simulink model "MIL_ASW"  (R2019b)
settings: Solver=FixedStepDiscrete  StartTime=0.0  StopTime=2  FixedStep=0.001  RelTol=1e-3  EnableMultiTasking=on
model workspace (MAT data in the model file):
  AccPedlCanVal = Simulink.Signal
  AccPedlCanVal.Description = 'the raw value of Engine Throttle from CAN, 0-255'
  AccPedlCanVal.DataType = 'uint8'
  AccPedlCanVal.Dimensions = -1
  AccPedlCanVal.DimensionsMode = 'auto'
  AccPedlCanVal.Complexity = 'auto'
  AccPedlCanVal.SampleTime = -1
  AccPedlCanVal.SamplingMode = 'auto'
  AccPedlVal = Simulink.Signal
  AccPedlVal.Description = 'the value of Engine Throttle percentage, 0-100'
  AccPedlVal.DataType = 'uint8'
  AccPedlVal.Dimensions = -1
  AccPedlVal.DimensionsMode = 'auto'
  AccPedlVal.Complexity = 'auto'
  AccPedlVal.SampleTime = -1
  AccPedlVal.SamplingMode = 'auto'
  BrkPedlCanVal = Simulink.Signal
  BrkPedlCanVal.Description = 'the raw value of Brake from CAN, 0-255'
  BrkPedlCanVal.DataType = 'uint8'
  BrkPedlCanVal.Dimensions = -1
  BrkPedlCanVal.DimensionsMode = 'auto'
  BrkPedlCanVal.Complexity = 'auto'
  BrkPedlCanVal.SampleTime = -1
  BrkPedlCanVal.SamplingMode = 'auto'
  BrkPedlVal = Simulink.Signal
  BrkPedlVal.Description = 'the value of Brake Pedal percentage, 0-100'
  BrkPedlVal.DataType = 'uint8'
  BrkPedlVal.Dimensions = -1
  BrkPedlVal.DimensionsMode = 'auto'
  BrkPedlVal.Complexity = 'auto'
  BrkPedlVal.SampleTime = -1
  BrkPedlVal.SamplingMode = 'auto'
  Cal1 = Simulink.Parameter
  Cal1.Value = 100
  Cal1.DataType = 'uint16'
  Cal1.Dimensions = [1 1]
  Cal10 = Simulink.Parameter
  Cal10.Value = 10
  Cal10.DataType = 'uint16'
  Cal10.Dimensions = [1 1]
  Cal11 = Simulink.Parameter
  Cal11.Value = 50
  Cal11.DataType = 'uint16'
  Cal11.Dimensions = [1 1]
  Cal12 = Simulink.Parameter
  Cal12.Value = 50
  Cal12.DataType = 'int16'
  Cal12.Dimensions = [1 1]
  Cal2 = Simulink.Parameter
  Cal2.Value = 10
  Cal2.DataType = 'uint16'
  Cal2.Dimensions = [1 1]
  Cal3 = Simulink.Parameter
  Cal3.Value = 200
  Cal3.DataType = 'uint16'
  Cal3.Dimensions = [1 1]
  Cal4 = Simulink.Parameter
  Cal4.Value = 50
  Cal4.DataType = 'int16'
  Cal4.Dimensions = [1 1]
  Cal5 = Simulink.Parameter
  Cal5.Value = 100
  Cal5.DataType = 'uint16'
  Cal5.Dimensions = [1 1]
  Cal6 = Simulink.Parameter
  Cal6.Value = 10
  Cal6.DataType = 'uint16'
  Cal6.Dimensions = [1 1]
  Cal7 = Simulink.Parameter
  Cal7.Value = 50
  Cal7.DataType = 'uint16'
  Cal7.Dimensions = [1 1]
  Cal8 = Simulink.Parameter
  Cal8.Value = 50
  Cal8.DataType = 'int16'
  Cal8.Dimensions = [1 1]
  Cal9 = Simulink.Parameter
  Cal9.Value = 100
  Cal9.DataType = 'uint16'
  Cal9.Dimensions = [1 1]
  Clu1Act = Simulink.Signal
  Clu1Act.DataType = 'uint8'
  Clu1Act.Dimensions = -1
  Clu1Act.DimensionsMode = 'auto'
  Clu1Act.Complexity = 'auto'
  Clu1Act.SampleTime = -1
  Clu1Act.SamplingMode = 'auto'
  Clu1PTar = Simulink.Signal
  Clu1PTar.DataType = 'uint16'
  Clu1PTar.Dimensions = -1
  Clu1PTar.DimensionsMode = 'auto'
  Clu1PTar.Complexity = 'auto'
  Clu1PTar.SampleTime = -1
  Clu1PTar.SamplingMode = 'auto'
  Clu1Req = Simulink.Signal
  Clu1Req.DataType = 'uint8'
  Clu1Req.Dimensions = -1
  Clu1Req.DimensionsMode = 'auto'
  Clu1Req.Complexity = 'auto'
  Clu1Req.SampleTime = -1
  Clu1Req.SamplingMode = 'auto'
  Clu1Req.InitialValue = '0'
  Clu1TqTar = Simulink.Signal
  Clu1TqTar.DataType = 'uint16'
  Clu1TqTar.Dimensions = -1
  Clu1TqTar.DimensionsMode = 'auto'
  Clu1TqTar.Complexity = 'auto'
  Clu1TqTar.SampleTime = -1
  Clu1TqTar.SamplingMode = 'auto'
  Clu2Act = Simulink.Signal
  Clu2Act.DataType = 'uint8'
  Clu2Act.Dimensions = -1
  Clu2Act.DimensionsMode = 'auto'
  Clu2Act.Complexity = 'auto'
  Clu2Act.SampleTime = -1
  Clu2Act.SamplingMode = 'auto'
  Clu2PTar = Simulink.Signal
  Clu2PTar.DataType = 'uint16'
  Clu2PTar.Dimensions = -1
  Clu2PTar.DimensionsMode = 'auto'
  Clu2PTar.Complexity = 'auto'
  Clu2PTar.SampleTime = -1
  Clu2PTar.SamplingMode = 'auto'
  Clu2Req = Simulink.Signal
  Clu2Req.DataType = 'uint8'
  Clu2Req.Dimensions = -1
  Clu2Req.DimensionsMode = 'auto'
  Clu2Req.Complexity = 'auto'
  Clu2Req.SampleTime = -1
  Clu2Req.SamplingMode = 'auto'
  Clu2Req.InitialValue = '0'
  Clu2TqTar = Simulink.Signal
  Clu2TqTar.DataType = 'uint16'
  Clu2TqTar.Dimensions = -1
  Clu2TqTar.DimensionsMode = 'auto'
  Clu2TqTar.Complexity = 'auto'
  Clu2TqTar.SampleTime = -1
  Clu2TqTar.SamplingMode = 'auto'
  CluKissPtPLnch = Simulink.Parameter
  CluKissPtPLnch.Value = 2200
  CluKissPtPLnch.DataType = 'uint16'
  CluKissPtPLnch.Dimensions = [1 1]
  CluOilTRawVal = Simulink.Signal
  CluOilTRawVal.Description = 'the raw value of Clutch oil temperature sensor, 0-255'
  CluOilTRawVal.DataType = 'uint16'
  CluOilTRawVal.Dimensions = -1
  CluOilTRawVal.DimensionsMode = 'auto'
  CluOilTRawVal.Complexity = 'auto'
  CluOilTRawVal.SampleTime = -1
  CluOilTRawVal.SamplingMode = 'auto'
  CluOilTVal = Simulink.Signal
  CluOilTVal.Description = 'the value of Clutch oil temperature'
  CluOilTVal.DataType = 'uint16'
  CluOilTVal.Dimensions = -1
  CluOilTVal.DimensionsMode = 'auto'
  CluOilTVal.Complexity = 'auto'
  CluOilTVal.SampleTime = -1
  CluOilTVal.SamplingMode = 'auto'
  CluOpenTqRatMax = Simulink.Parameter
  CluOpenTqRatMax.Value = 100
  CluOpenTqRatMax.DataType = 'uint16'
  CluOpenTqRatMax.Dimensions = [1 1]
  CluPMap = Simulink.Parameter
  CluPMap.Value = [0 1300 9000]
  CluPMap.DataType = 'uint16'
  CluPMap.Dimensions = [1 3]
  CluPMax = Simulink.Parameter
  CluPMax.Value = 600
  CluPMax.DataType = 'uint16'
  CluPMax.Dimensions = [1 1]
  CluPMaxGear1 = Simulink.Parameter
  CluPMaxGear1.Value = 4000
  CluPMaxGear1.DataType = 'uint16'
  CluPMaxGear1.Dimensions = [1 1]
  CluPMaxGear2 = Simulink.Parameter
  CluPMaxGear2.Value = 4500
  CluPMaxGear2.DataType = 'uint16'
  CluPMaxGear2.Dimensions = [1 1]
  CluPMaxGear3 = Simulink.Parameter
  CluPMaxGear3.Value = 5000
  CluPMaxGear3.DataType = 'uint16'
  CluPMaxGear3.Dimensions = [1 1]
  CluPMaxGear4 = Simulink.Parameter
  CluPMaxGear4.Value = 5500
  CluPMaxGear4.DataType = 'uint16'
  CluPMaxGear4.Dimensions = [1 1]
  CluPMaxGear5 = Simulink.Parameter
  CluPMaxGear5.Value = 6000
  CluPMaxGear5.DataType = 'uint16'
  CluPMaxGear5.Dimensions = [1 1]
  CluPMaxGear6 = Simulink.Parameter
  CluPMaxGear6.Value = 6000
  CluPMaxGear6.DataType = 'uint16'
  CluPMaxGear6.Dimensions = [1 1]
  CluPMaxGearR = Simulink.Parameter
  CluPMaxGearR.Value = 3500
  CluPMaxGearR.DataType = 'uint16'
  CluPMaxGearR.Dimensions = [1 1]
  CluPMin = Simulink.Parameter
  CluPMin.Value = 1300
  CluPMin.DataType = 'uint16'
  CluPMin.Dimensions = [1 1]
  CluPosnMax = Simulink.Parameter
  CluPosnMax.Value = 4550
  CluPosnMax.DataType = 'uint16'
  CluPosnMax.Dimensions = [1 1]
  CluSoln1IRawVal = Simulink.Signal
  CluSoln1IRawVal.DataType = 'uint16'
  CluSoln1IRawVal.Dimensions = -1
  CluSoln1IRawVal.DimensionsMode = 'auto'
  CluSoln1IRawVal.Complexity = 'auto'
  CluSoln1IRawVal.SampleTime = -1
  CluSoln1IRawVal.SamplingMode = 'auto'
  CluSoln1IReq = Simulink.Signal
  CluSoln1IReq.DataType = 'uint16'
  CluSoln1IReq.Dimensions = -1
  CluSoln1IReq.DimensionsMode = 'auto'
  CluSoln1IReq.Complexity = 'auto'
  CluSoln1IReq.SampleTime = -1
  CluSoln1IReq.SamplingMode = 'auto'
  CluSoln1IReqFlg = Simulink.Signal
  CluSoln1IReqFlg.DataType = 'uint8'
  CluSoln1IReqFlg.Dimensions = -1
  CluSoln1IReqFlg.DimensionsMode = 'auto'
  CluSoln1IReqFlg.Complexity = 'auto'
  CluSoln1IReqFlg.SampleTime = -1
  CluSoln1IReqFlg.SamplingMode = 'auto'
  CluSoln1IVal = Simulink.Signal
  CluSoln1IVal.DataType = 'uint16'
  CluSoln1IVal.Dimensions = -1
  CluSoln1IVal.DimensionsMode = 'auto'
  CluSoln1IVal.Complexity = 'auto'
  CluSoln1IVal.SampleTime = -1
  CluSoln1IVal.SamplingMode = 'auto'
  CluSoln1LineI = Simulink.Parameter
  CluSoln1LineI.Value = [0 200 400 600 800 950]
  CluSoln1LineI.DataType = 'uint16'
  CluSoln1LineI.Dimensions = [1 6]
  CluSoln1LineP = Simulink.Parameter
  CluSoln1LineP.Value = [0 1 2500 8850 15770 20000]
  CluSoln1LineP.DataType = 'uint16'
  CluSoln1LineP.Dimensions = [1 6]
  CluSoln1Pwm = Simulink.Signal
  CluSoln1Pwm.DataType = 'uint16'
  CluSoln1Pwm.Dimensions = -1
  CluSoln1Pwm.DimensionsMode = 'auto'
  CluSoln1Pwm.Complexity = 'auto'
  CluSoln1Pwm.SampleTime = -1
  CluSoln1Pwm.SamplingMode = 'auto'
  CluSoln2IRawVal = Simulink.Signal
  CluSoln2IRawVal.DataType = 'uint16'
  CluSoln2IRawVal.Dimensions = -1
  CluSoln2IRawVal.DimensionsMode = 'auto'
  CluSoln2IRawVal.Complexity = 'auto'
  CluSoln2IRawVal.SampleTime = -1
  CluSoln2IRawVal.SamplingMode = 'auto'
  CluSoln2IReq = Simulink.Signal
  CluSoln2IReq.DataType = 'uint16'
  CluSoln2IReq.Dimensions = -1
  CluSoln2IReq.DimensionsMode = 'auto'
  CluSoln2IReq.Complexity = 'auto'
  CluSoln2IReq.SampleTime = -1
  CluSoln2IReq.SamplingMode = 'auto'
  CluSoln2IReqFlg = Simulink.Signal
  CluSoln2IReqFlg.DataType = 'uint8'
  CluSoln2IReqFlg.Dimensions = -1
  CluSoln2IReqFlg.DimensionsMode = 'auto'
  CluSoln2IReqFlg.Complexity = 'auto'
  CluSoln2IReqFlg.SampleTime = -1
  CluSoln2IReqFlg.SamplingMode = 'auto'
  CluSoln2IVal = Simulink.Signal
  CluSoln2IVal.DataType = 'uint16'
  CluSoln2IVal.Dimensions = -1
  CluSoln2IVal.DimensionsMode = 'auto'
  CluSoln2IVal.Complexity = 'auto'
  CluSoln2IVal.SampleTime = -1
  CluSoln2IVal.SamplingMode = 'auto'
  CluSoln2LineI = Simulink.Parameter
  CluSoln2LineI.Value = [0 200 400 600 800 950]
  CluSoln2LineI.DataType = 'uint16'
  CluSoln2LineI.Dimensions = [1 6]
  CluSoln2LineP = Simulink.Parameter
  CluSoln2LineP.Value = [0 1 2500 8850 15770 20000]
  CluSoln2LineP.DataType = 'uint16'
  CluSoln2LineP.Dimensions = [1 6]
  CluSoln2Pwm = Simulink.Signal
  CluSoln2Pwm.DataType = 'uint16'
  CluSoln2Pwm.Dimensions = -1
  CluSoln2Pwm.DimensionsMode = 'auto'
  CluSoln2Pwm.Complexity = 'auto'
  CluSoln2Pwm.SampleTime = -1
  CluSoln2Pwm.SamplingMode = 'auto'
  CluTqMap = Simulink.Parameter
  CluTqMap.Value = [0 1 35000]
  CluTqMap.DataType = 'uint16'
  CluTqMap.Dimensions = [1 3]
  CrnkSpdRawVal = Simulink.Signal
  CrnkSpdRawVal.Description = 'the raw value of the frequency of crank shaft signal, Hz'
  CrnkSpdRawVal.DataType = 'uint16'
  CrnkSpdRawVal.Dimensions = -1
  CrnkSpdRawVal.DimensionsMode = 'auto'
  CrnkSpdRawVal.Complexity = 'auto'
  CrnkSpdRawVal.SampleTime = -1
  CrnkSpdRawVal.SamplingMode = 'auto'
  CrnkSpdVal = Simulink.Signal
  CrnkSpdVal.Description = 'the value of enigne crank shaft speed, rpm'
  CrnkSpdVal.DataType = 'uint16'
  CrnkSpdVal.Dimensions = -1
  CrnkSpdVal.DimensionsMode = 'auto'
  CrnkSpdVal.Complexity = 'auto'
  CrnkSpdVal.SampleTime = -1
  CrnkSpdVal.SamplingMode = 'auto'
  Drive_Intensity_Fuzzy.name = 'Launch_Intensity_Fuzzy'
  Drive_Intensity_Fuzzy.type = 'mamdani'
  Drive_Intensity_Fuzzy.andMethod = 'min'
  Drive_Intensity_Fuzzy.orMethod = 'max'
  Drive_Intensity_Fuzzy.defuzzMethod = 'centroid'
  Drive_Intensity_Fuzzy.impMethod = 'min'
  Drive_Intensity_Fuzzy.aggMethod = 'max'
  Drive_Intensity_Fuzzy.input(1).name = 'Pedl'
  Drive_Intensity_Fuzzy.input(1).range = [0 100]
  Drive_Intensity_Fuzzy.input(1).mf(1).name = 'VS'
  Drive_Intensity_Fuzzy.input(1).mf(1).type = 'trimf'
  Drive_Intensity_Fuzzy.input(1).mf(1).params = [0 0 25]
  Drive_Intensity_Fuzzy.input(1).mf(2).name = 'S'
  Drive_Intensity_Fuzzy.input(1).mf(2).type = 'trimf'
  Drive_Intensity_Fuzzy.input(1).mf(2).params = [0 25 50]
  Drive_Intensity_Fuzzy.input(1).mf(3).name = 'M'
  Drive_Intensity_Fuzzy.input(1).mf(3).type = 'trimf'
  Drive_Intensity_Fuzzy.input(1).mf(3).params = [25 50 75]
  Drive_Intensity_Fuzzy.input(1).mf(4).name = 'B'
  Drive_Intensity_Fuzzy.input(1).mf(4).type = 'trimf'
  Drive_Intensity_Fuzzy.input(1).mf(4).params = [50 75 100]
  Drive_Intensity_Fuzzy.input(1).mf(5).name = 'VB'
  Drive_Intensity_Fuzzy.input(1).mf(5).type = 'trimf'
  Drive_Intensity_Fuzzy.input(1).mf(5).params = [75 100 110]
  Drive_Intensity_Fuzzy.input(2).name = 'dPedl'
  Drive_Intensity_Fuzzy.input(2).range = [-300 300]
  Drive_Intensity_Fuzzy.input(2).mf(1).name = 'NB'
  Drive_Intensity_Fuzzy.input(2).mf(1).type = 'trimf'
  Drive_Intensity_Fuzzy.input(2).mf(1).params = [-300 -300 -100]
  Drive_Intensity_Fuzzy.input(2).mf(2).name = 'NS'
  Drive_Intensity_Fuzzy.input(2).mf(2).type = 'trimf'
  Drive_Intensity_Fuzzy.input(2).mf(2).params = [-300 -100 0]
  Drive_Intensity_Fuzzy.input(2).mf(3).name = 'Z'
  Drive_Intensity_Fuzzy.input(2).mf(3).type = 'trimf'
  Drive_Intensity_Fuzzy.input(2).mf(3).params = [-100 0 100]
  Drive_Intensity_Fuzzy.input(2).mf(4).name = 'PS'
  Drive_Intensity_Fuzzy.input(2).mf(4).type = 'trimf'
  Drive_Intensity_Fuzzy.input(2).mf(4).params = [0 100 200]
  Drive_Intensity_Fuzzy.input(2).mf(5).name = 'PM'
  Drive_Intensity_Fuzzy.input(2).mf(5).type = 'trimf'
  Drive_Intensity_Fuzzy.input(2).mf(5).params = [100 200 300]
  Drive_Intensity_Fuzzy.input(2).mf(6).name = 'PB'
  Drive_Intensity_Fuzzy.input(2).mf(6).type = 'trimf'
  Drive_Intensity_Fuzzy.input(2).mf(6).params = [200 300 350]
  Drive_Intensity_Fuzzy.output.name = 'Inten'
  Drive_Intensity_Fuzzy.output.range = [0 100]
  Drive_Intensity_Fuzzy.output.mf(1).name = 'VS'
  Drive_Intensity_Fuzzy.output.mf(1).type = 'trimf'
  Drive_Intensity_Fuzzy.output.mf(1).params = [0 0 25]
  Drive_Intensity_Fuzzy.output.mf(2).name = 'S'
  Drive_Intensity_Fuzzy.output.mf(2).type = 'trimf'
  Drive_Intensity_Fuzzy.output.mf(2).params = [0 25 50]
  Drive_Intensity_Fuzzy.output.mf(3).name = 'M'
  Drive_Intensity_Fuzzy.output.mf(3).type = 'trimf'
  Drive_Intensity_Fuzzy.output.mf(3).params = [25 50 75]
  Drive_Intensity_Fuzzy.output.mf(4).name = 'F'
  Drive_Intensity_Fuzzy.output.mf(4).type = 'trimf'
  Drive_Intensity_Fuzzy.output.mf(4).params = [50 75 100]
  Drive_Intensity_Fuzzy.output.mf(5).name = 'VF'
  Drive_Intensity_Fuzzy.output.mf(5).type = 'trimf'
  Drive_Intensity_Fuzzy.output.mf(5).params = [75 100 110]
  Drive_Intensity_Fuzzy.rule(1).antecedent = [1 1]
  Drive_Intensity_Fuzzy.rule(1).consequent = 1
  Drive_Intensity_Fuzzy.rule(1).weight = 1
  Drive_Intensity_Fuzzy.rule(1).connection = 1
  Drive_Intensity_Fuzzy.rule(2).antecedent = [1 2]
  Drive_Intensity_Fuzzy.rule(2).consequent = 1
  Drive_Intensity_Fuzzy.rule(2).weight = 1
  Drive_Intensity_Fuzzy.rule(2).connection = 1
  Drive_Intensity_Fuzzy.rule(3).antecedent = [1 3]
  Drive_Intensity_Fuzzy.rule(3).consequent = 1
  Drive_Intensity_Fuzzy.rule(3).weight = 1
  Drive_Intensity_Fuzzy.rule(3).connection = 1
  Drive_Intensity_Fuzzy.rule(4).antecedent = [1 4]
  Drive_Intensity_Fuzzy.rule(4).consequent = 2
  Drive_Intensity_Fuzzy.rule(4).weight = 1
  Drive_Intensity_Fuzzy.rule(4).connection = 1
  Drive_Intensity_Fuzzy.rule(5).antecedent = [1 5]
  Drive_Intensity_Fuzzy.rule(5).consequent = 3
  Drive_Intensity_Fuzzy.rule(5).weight = 1
  Drive_Intensity_Fuzzy.rule(5).connection = 1
  Drive_Intensity_Fuzzy.rule(6).antecedent = [1 6]
  Drive_Intensity_Fuzzy.rule(6).consequent = 4
  Drive_Intensity_Fuzzy.rule(6).weight = 1
  Drive_Intensity_Fuzzy.rule(6).connection = 1
  Drive_Intensity_Fuzzy.rule(7).antecedent = [2 1]
  Drive_Intensity_Fuzzy.rule(7).consequent = 1
  Drive_Intensity_Fuzzy.rule(7).weight = 1
  Drive_Intensity_Fuzzy.rule(7).connection = 1
  Drive_Intensity_Fuzzy.rule(8).antecedent = [2 2]
  Drive_Intensity_Fuzzy.rule(8).consequent = 2
  Drive_Intensity_Fuzzy.rule(8).weight = 1
  Drive_Intensity_Fuzzy.rule(8).connection = 1
  Drive_Intensity_Fuzzy.rule(9).antecedent = [2 3]
  Drive_Intensity_Fuzzy.rule(9).consequent = 2
  Drive_Intensity_Fuzzy.rule(9).weight = 1
  Drive_Intensity_Fuzzy.rule(9).connection = 1
  Drive_Intensity_Fuzzy.rule(10).antecedent = [2 4]
  Drive_Intensity_Fuzzy.rule(10).consequent = 3
  Drive_Intensity_Fuzzy.rule(10).weight = 1
  Drive_Intensity_Fuzzy.rule(10).connection = 1
  Drive_Intensity_Fuzzy.rule(11).antecedent = [2 5]
  Drive_Intensity_Fuzzy.rule(11).consequent = 4
  Drive_Intensity_Fuzzy.rule(11).weight = 1
  Drive_Intensity_Fuzzy.rule(11).connection = 1
  Drive_Intensity_Fuzzy.rule(12).antecedent = [2 6]
  Drive_Intensity_Fuzzy.rule(12).consequent = 4
  Drive_Intensity_Fuzzy.rule(12).weight = 1
  Drive_Intensity_Fuzzy.rule(12).connection = 1
  Drive_Intensity_Fuzzy.rule(13).antecedent = [3 1]
  Drive_Intensity_Fuzzy.rule(13).consequent = 1
  Drive_Intensity_Fuzzy.rule(13).weight = 1
  Drive_Intensity_Fuzzy.rule(13).connection = 1
  Drive_Intensity_Fuzzy.rule(14).antecedent = [3 2]
  Drive_Intensity_Fuzzy.rule(14).consequent = 2
  Drive_Intensity_Fuzzy.rule(14).weight = 1
  Drive_Intensity_Fuzzy.rule(14).connection = 1
  Drive_Intensity_Fuzzy.rule(15).antecedent = [3 3]
  Drive_Intensity_Fuzzy.rule(15).consequent = 3
  Drive_Intensity_Fuzzy.rule(15).weight = 1
  Drive_Intensity_Fuzzy.rule(15).connection = 1
  Drive_Intensity_Fuzzy.rule(16).antecedent = [3 4]
  Drive_Intensity_Fuzzy.rule(16).consequent = 4
  Drive_Intensity_Fuzzy.rule(16).weight = 1
  Drive_Intensity_Fuzzy.rule(16).connection = 1
  Drive_Intensity_Fuzzy.rule(17).antecedent = [3 5]
  Drive_Intensity_Fuzzy.rule(17).consequent = 5
  Drive_Intensity_Fuzzy.rule(17).weight = 1
  Drive_Intensity_Fuzzy.rule(17).connection = 1
  Drive_Intensity_Fuzzy.rule(18).antecedent = [3 6]
  Drive_Intensity_Fuzzy.rule(18).consequent = 5
  Drive_Intensity_Fuzzy.rule(18).weight = 1
  Drive_Intensity_Fuzzy.rule(18).connection = 1
  Drive_Intensity_Fuzzy.rule(19).antecedent = [4 1]
  Drive_Intensity_Fuzzy.rule(19).consequent = 1
  Drive_Intensity_Fuzzy.rule(19).weight = 1
  Drive_Intensity_Fuzzy.rule(19).connection = 1
  Drive_Intensity_Fuzzy.rule(20).antecedent = [4 2]
  Drive_Intensity_Fuzzy.rule(20).consequent = 2
  Drive_Intensity_Fuzzy.rule(20).weight = 1
  Drive_Intensity_Fuzzy.rule(20).connection = 1
  Drive_Intensity_Fuzzy.rule(21).antecedent = [4 3]
  Drive_Intensity_Fuzzy.rule(21).consequent = 4
  Drive_Intensity_Fuzzy.rule(21).weight = 1
  Drive_Intensity_Fuzzy.rule(21).connection = 1
  Drive_Intensity_Fuzzy.rule(22).antecedent = [4 4]
  Drive_Intensity_Fuzzy.rule(22).consequent = 4
  Drive_Intensity_Fuzzy.rule(22).weight = 1
  Drive_Intensity_Fuzzy.rule(22).connection = 1
  Drive_Intensity_Fuzzy.rule(23).antecedent = [4 5]
  Drive_Intensity_Fuzzy.rule(23).consequent = 5
  Drive_Intensity_Fuzzy.rule(23).weight = 1
  Drive_Intensity_Fuzzy.rule(23).connection = 1
  Drive_Intensity_Fuzzy.rule(24).antecedent = [4 6]
  Drive_Intensity_Fuzzy.rule(24).consequent = 5
  Drive_Intensity_Fuzzy.rule(24).weight = 1
  Drive_Intensity_Fuzzy.rule(24).connection = 1
  Drive_Intensity_Fuzzy.rule(25).antecedent = [5 1]
  Drive_Intensity_Fuzzy.rule(25).consequent = 1
  Drive_Intensity_Fuzzy.rule(25).weight = 1
  Drive_Intensity_Fuzzy.rule(25).connection = 1
  Drive_Intensity_Fuzzy.rule(26).antecedent = [5 2]
  Drive_Intensity_Fuzzy.rule(26).consequent = 2
  Drive_Intensity_Fuzzy.rule(26).weight = 1
  Drive_Intensity_Fuzzy.rule(26).connection = 1
  Drive_Intensity_Fuzzy.rule(27).antecedent = [5 3]
  Drive_Intensity_Fuzzy.rule(27).consequent = 5
  Drive_Intensity_Fuzzy.rule(27).weight = 1
  Drive_Intensity_Fuzzy.rule(27).connection = 1
  Drive_Intensity_Fuzzy.rule(28).antecedent = [5 4]
  Drive_Intensity_Fuzzy.rule(28).consequent = 5
  Drive_Intensity_Fuzzy.rule(28).weight = 1
  Drive_Intensity_Fuzzy.rule(28).connection = 1
  Drive_Intensity_Fuzzy.rule(29).antecedent = [5 5]
  Drive_Intensity_Fuzzy.rule(29).consequent = 5
  Drive_Intensity_Fuzzy.rule(29).weight = 1
  Drive_Intensity_Fuzzy.rule(29).connection = 1
  Drive_Intensity_Fuzzy.rule(30).antecedent = [5 6]
  Drive_Intensity_Fuzzy.rule(30).consequent = 5
  Drive_Intensity_Fuzzy.rule(30).weight = 1
  Drive_Intensity_Fuzzy.rule(30).connection = 1
  DrvIntenFzzy = Simulink.LookupTable
  DrvIntenFzzy.Table = Simulink.lookuptable.Table
  DrvIntenFzzy.Table.Value = [8  9  9  8  9  19  25  41  59  75; 9  20  21  21  21  31  36  52  61  75; 8  19  24  25  25  34  46  62  71  75; 9  19  24  25  34  45  59  67  76  76; 8  19  24  25  41  52  68  72  83  83; 8  19  24  25  48  59  75  81  91  92; 9  19  24  25  55  66  75  81  91  91; 8  19  24  25  56  75  75  81  91  92; 9  20  23  25  58  79  79  80  91  91; 8  19  24  25  55  91  92  91  91  92]
  DrvIntenFzzy.Table.Dimensions = [10 10]
  DrvIntenFzzy.Table.DataType = 'int16'
  DrvIntenFzzy.Table.FieldName = 'Table'
  DrvIntenFzzy.Breakpoints(1) = Simulink.lookuptable.Breakpoint
  DrvIntenFzzy.Breakpoints(1).Value = [0 11 22 33 44 56 67 78 89 100]
  DrvIntenFzzy.Breakpoints(1).TunableSizeName = 'N1'
  DrvIntenFzzy.Breakpoints(1).Dimensions = [1 10]
  DrvIntenFzzy.Breakpoints(1).DataType = 'int16'
  DrvIntenFzzy.Breakpoints(1).FieldName = 'BP1'
  DrvIntenFzzy.Breakpoints(2) = Simulink.lookuptable.Breakpoint
  DrvIntenFzzy.Breakpoints(2).Value = [-300 -233 -167 -100 -33 33 100 167 233 300]
  DrvIntenFzzy.Breakpoints(2).TunableSizeName = 'N2'
  DrvIntenFzzy.Breakpoints(2).Dimensions = [1 10]
  DrvIntenFzzy.Breakpoints(2).DataType = 'int16'
  DrvIntenFzzy.Breakpoints(2).FieldName = 'BP2'
  DrvIntenFzzy.SupportTunableSize = 0
  DrvIntenFzzy.StructTypeInfo = Simulink.lookuptable.StructTypeInfo
  DrvIntenFzzy.StructTypeInfo.Name = 'DrvIntenFzzyStruct'
  DrvIntenFzzy.StructTypeInfo.DataScope = 'Auto'
  EngNIdle = Simulink.Parameter
  EngNIdle.Value = 750
  EngNIdle.DataType = 'uint16'
  EngNIdle.Dimensions = [1 1]
  EngNIdleMin = Simulink.Parameter
  EngNIdleMin.Value = 400
  EngNIdleMin.DataType = 'uint16'
  EngNIdleMin.Dimensions = [1 1]
  EngSpdCanVal = Simulink.Signal
  EngSpdCanVal.Description = 'engine speed information from CAN bus'
  EngSpdCanVal.DataType = 'uint16'
  EngSpdCanVal.Dimensions = -1
  EngSpdCanVal.DimensionsMode = 'auto'
  EngSpdCanVal.Complexity = 'auto'
  EngSpdCanVal.SampleTime = -1
  EngSpdCanVal.SamplingMode = 'auto'
  EngThrCanVal = Simulink.Signal
  EngThrCanVal.Description = 'engine throttle opening information from CAN bus'
  EngThrCanVal.DataType = 'uint8'
  EngThrCanVal.Dimensions = -1
  EngThrCanVal.DimensionsMode = 'auto'
  EngThrCanVal.Complexity = 'auto'
  EngThrCanVal.SampleTime = -1
  EngThrCanVal.SamplingMode = 'auto'
  EngTqAdd = Simulink.Parameter
  EngTqAdd.Value = 2500
  EngTqAdd.DataType = 'uint16'
  EngTqAdd.Dimensions = [1 1]
  EngTqCanVal = Simulink.Signal
  EngTqCanVal.Description = 'engine torque information from CAN bus'
  EngTqCanVal.DataType = 'uint16'
  EngTqCanVal.Dimensions = -1
  EngTqCanVal.DimensionsMode = 'auto'
  EngTqCanVal.Complexity = 'auto'
  EngTqCanVal.SampleTime = -1
  EngTqCanVal.SamplingMode = 'auto'
  EngTqIntvFlg = Simulink.Signal
  EngTqIntvFlg.DataType = 'uint8'
  EngTqIntvFlg.Dimensions = -1
  EngTqIntvFlg.DimensionsMode = 'auto'
  EngTqIntvFlg.Complexity = 'auto'
  EngTqIntvFlg.SampleTime = -1
  EngTqIntvFlg.SamplingMode = 'auto'
  EngTqIntvRat = Simulink.Signal
  EngTqIntvRat.DataType = 'uint8'
  EngTqIntvRat.Dimensions = -1
  EngTqIntvRat.DimensionsMode = 'auto'
  EngTqIntvRat.Complexity = 'auto'
  EngTqIntvRat.SampleTime = -1
  EngTqIntvRat.SamplingMode = 'auto'
  EngTqMapExtChartc = Simulink.Parameter
  EngTqMapExtChartc.Value = [0 0 11817 21322 25300 28928 30352 32100 33708 35000 35000 35000 35000 35000 33732 32308 30670 26743 22827 14400 0]
  EngTqMapExtChartc.DataType = 'uint16'
  EngTqMapExtChartc.Dimensions = [1 21]
  EngTqMapSpdIndx = Simulink.Parameter
  EngTqMapSpdIndx.Value = [0 400 517 633 750 1107 1463 1820 2177 2533 2890 3247 3603 3960 4317 4673 5030 5387 5743 6100 6500]
  EngTqMapSpdIndx.DataType = 'uint16'
  EngTqMapSpdIndx.Dimensions = [1 21]
  EngTqMapThrtIndx = Simulink.Parameter
  EngTqMapThrtIndx.Value = [0 10 20 30 40 50 60 70 80 90 100]
  EngTqMapThrtIndx.DataType = 'uint8'
  EngTqMapThrtIndx.Dimensions = [1 11]
  EngTqMapTqMax = Simulink.Parameter
  EngTqMapTqMax.Value = [4179 4179 13259 23544 26944 29368 32550 33431 34042 34548 35000]
  EngTqMapTqMax.DataType = 'uint16'
  EngTqMapTqMax.Dimensions = [1 11]
  EngTqMaxNorm = Simulink.Parameter
  EngTqMaxNorm.Value = 35000
  EngTqMaxNorm.DataType = 'uint16'
  EngTqMaxNorm.Dimensions = [1 1]
  EngTqRef = Simulink.Parameter
  EngTqRef.Value = 250
  EngTqRef.DataType = 'uint16'
  EngTqRef.Dimensions = [1 1]
  EvenCluPRawVal = Simulink.Signal
  EvenCluPRawVal.Description = ' the raw value of Even Gear Clutch Pressure sensor, 0-255'
  EvenCluPRawVal.DataType = 'uint16'
  EvenCluPRawVal.Dimensions = -1
  EvenCluPRawVal.DimensionsMode = 'auto'
  EvenCluPRawVal.Complexity = 'auto'
  EvenCluPRawVal.SampleTime = -1
  EvenCluPRawVal.SamplingMode = 'auto'
  EvenCluPVal = Simulink.Signal
  EvenCluPVal.Description = 'the value of Even Gear Clutch Pressure sensor *10, Bar'
  EvenCluPVal.DataType = 'uint16'
  EvenCluPVal.Dimensions = -1
  EvenCluPVal.DimensionsMode = 'auto'
  EvenCluPVal.Complexity = 'auto'
  EvenCluPVal.SampleTime = -1
  EvenCluPVal.SamplingMode = 'auto'
  EvenInpSpdRawVal = Simulink.Signal
  EvenInpSpdRawVal.Description = 'the raw value of the frequency of even input shaft signal, Hz'
  EvenInpSpdRawVal.DataType = 'uint16'
  EvenInpSpdRawVal.Dimensions = -1
  EvenInpSpdRawVal.DimensionsMode = 'auto'
  EvenInpSpdRawVal.Complexity = 'auto'
  EvenInpSpdRawVal.SampleTime = -1
  EvenInpSpdRawVal.SamplingMode = 'auto'
  EvenInpSpdVal = Simulink.Signal
  EvenInpSpdVal.Description = 'the value of even input shaft speed, rpm'
  EvenInpSpdVal.DataType = 'uint16'
  EvenInpSpdVal.Dimensions = -1
  EvenInpSpdVal.DimensionsMode = 'auto'
  EvenInpSpdVal.Complexity = 'auto'
  EvenInpSpdVal.SampleTime = -1
  EvenInpSpdVal.SamplingMode = 'auto'
  FcnCallTime = Simulink.Parameter
  FcnCallTime.Value = 10
  FcnCallTime.DataType = 'uint8'
  FcnCallTime.Dimensions = [1 1]
  FinalRat = Simulink.Parameter
  FinalRat.Value = [428 285]
  FinalRat.DataType = 'uint16'
  FinalRat.Dimensions = [1 2]
  Fork1A = Simulink.Parameter
  Fork1A.Value = 1
  Fork1A.DataType = 'uint8'
  Fork1A.Dimensions = [1 1]
  Fork1Act = Simulink.Signal
  Fork1Act.DataType = 'uint8'
  Fork1Act.Dimensions = -1
  Fork1Act.DimensionsMode = 'auto'
  Fork1Act.Complexity = 'auto'
  Fork1Act.SampleTime = -1
  Fork1Act.SamplingMode = 'auto'
  Fork1B = Simulink.Parameter
  Fork1B.Value = 3
  Fork1B.DataType = 'uint8'
  Fork1B.Dimensions = [1 1]
  Fork1DeltaSpdTar = Simulink.Parameter
  Fork1DeltaSpdTar.Value = 20
  Fork1DeltaSpdTar.DataType = 'uint16'
  Fork1DeltaSpdTar.Dimensions = [1 1]
  Fork1MaxSpd1A = Simulink.Parameter
  Fork1MaxSpd1A.Value = 4400
  Fork1MaxSpd1A.DataType = 'uint16'
  Fork1MaxSpd1A.Dimensions = [1 1]
  Fork1MaxSpd1B = Simulink.Parameter
  Fork1MaxSpd1B.Value = 4400
  Fork1MaxSpd1B.DataType = 'uint16'
  Fork1MaxSpd1B.Dimensions = [1 1]
  Fork1MaxSpd2A = Simulink.Parameter
  Fork1MaxSpd2A.Value = 3400
  Fork1MaxSpd2A.DataType = 'uint16'
  Fork1MaxSpd2A.Dimensions = [1 1]
  Fork1MaxSpd2B = Simulink.Parameter
  Fork1MaxSpd2B.Value = 3400
  Fork1MaxSpd2B.DataType = 'uint16'
  Fork1MaxSpd2B.Dimensions = [1 1]
  Fork1PosnA = Simulink.Parameter
  Fork1PosnA.Value = 795
  Fork1PosnA.DataType = 'uint16'
  Fork1PosnA.Dimensions = [1 1]
  Fork1PosnB = Simulink.Parameter
  Fork1PosnB.Value = 249
  Fork1PosnB.DataType = 'uint16'
  Fork1PosnB.Dimensions = [1 1]
  Fork1PosnMaxSpd1A = Simulink.Parameter
  Fork1PosnMaxSpd1A.Value = 560
  Fork1PosnMaxSpd1A.DataType = 'uint16'
  Fork1PosnMaxSpd1A.Dimensions = [1 1]
  Fork1PosnMaxSpd1B = Simulink.Parameter
  Fork1PosnMaxSpd1B.Value = 480
  Fork1PosnMaxSpd1B.DataType = 'uint16'
  Fork1PosnMaxSpd1B.Dimensions = [1 1]
  Fork1PosnMaxSpd2A = Simulink.Parameter
  Fork1PosnMaxSpd2A.Value = 720
  Fork1PosnMaxSpd2A.DataType = 'uint16'
  Fork1PosnMaxSpd2A.Dimensions = [1 1]
  Fork1PosnMaxSpd2B = Simulink.Parameter
  Fork1PosnMaxSpd2B.Value = 320
  Fork1PosnMaxSpd2B.DataType = 'uint16'
  Fork1PosnMaxSpd2B.Dimensions = [1 1]
  Fork1PosnNeut = Simulink.Parameter
  Fork1PosnNeut.Value = 513
  Fork1PosnNeut.DataType = 'uint16'
  Fork1PosnNeut.Dimensions = [1 1]
  Fork1PosnNeutA = Simulink.Parameter
  Fork1PosnNeutA.Value = 523
  Fork1PosnNeutA.DataType = 'uint16'
  Fork1PosnNeutA.Dimensions = [1 1]
  Fork1PosnNeutB = Simulink.Parameter
  Fork1PosnNeutB.Value = 503
  Fork1PosnNeutB.DataType = 'uint16'
  Fork1PosnNeutB.Dimensions = [1 1]
  Fork1PosnRawVal = Simulink.Signal
  Fork1PosnRawVal.Description = 'the raw value of the duty of fork 13 position pwm signal, 0-100'
  Fork1PosnRawVal.DataType = 'uint16'
  Fork1PosnRawVal.Dimensions = -1
  Fork1PosnRawVal.DimensionsMode = 'auto'
  Fork1PosnRawVal.Complexity = 'auto'
  Fork1PosnRawVal.SampleTime = -1
  Fork1PosnRawVal.SamplingMode = 'auto'
  Fork1PosnSyncA = Simulink.Parameter
  Fork1PosnSyncA.Value = 630
  Fork1PosnSyncA.DataType = 'uint16'
  Fork1PosnSyncA.Dimensions = [1 1]
  Fork1PosnSyncB = Simulink.Parameter
  Fork1PosnSyncB.Value = 410
  Fork1PosnSyncB.DataType = 'uint16'
  Fork1PosnSyncB.Dimensions = [1 1]
  Fork1PosnVal = Simulink.Signal
  Fork1PosnVal.Description = 'the value of fork 13 position, 0-100'
  Fork1PosnVal.DataType = 'uint16'
  Fork1PosnVal.Dimensions = -1
  Fork1PosnVal.DimensionsMode = 'auto'
  Fork1PosnVal.Complexity = 'auto'
  Fork1PosnVal.SampleTime = -1
  Fork1PosnVal.SamplingMode = 'auto'
  Fork1SyncTar = Simulink.Parameter
  Fork1SyncTar.Value = 20
  Fork1SyncTar.DataType = 'uint16'
  Fork1SyncTar.Dimensions = [1 1]
  Fork2A = Simulink.Parameter
  Fork2A.Value = 2
  Fork2A.DataType = 'uint8'
  Fork2A.Dimensions = [1 1]
  Fork2Act = Simulink.Signal
  Fork2Act.DataType = 'uint8'
  Fork2Act.Dimensions = -1
  Fork2Act.DimensionsMode = 'auto'
  Fork2Act.Complexity = 'auto'
  Fork2Act.SampleTime = -1
  Fork2Act.SamplingMode = 'auto'
  Fork2B = Simulink.Parameter
  Fork2B.Value = 4
  Fork2B.DataType = 'uint8'
  Fork2B.Dimensions = [1 1]
  Fork2DeltaSpdTar = Simulink.Parameter
  Fork2DeltaSpdTar.Value = 20
  Fork2DeltaSpdTar.DataType = 'uint16'
  Fork2DeltaSpdTar.Dimensions = [1 1]
  Fork2MaxSpd1A = Simulink.Parameter
  Fork2MaxSpd1A.Value = 4400
  Fork2MaxSpd1A.DataType = 'uint16'
  Fork2MaxSpd1A.Dimensions = [1 1]
  Fork2MaxSpd1B = Simulink.Parameter
  Fork2MaxSpd1B.Value = 4400
  Fork2MaxSpd1B.DataType = 'uint16'
  Fork2MaxSpd1B.Dimensions = [1 1]
  Fork2MaxSpd2A = Simulink.Parameter
  Fork2MaxSpd2A.Value = 3400
  Fork2MaxSpd2A.DataType = 'uint16'
  Fork2MaxSpd2A.Dimensions = [1 1]
  Fork2MaxSpd2B = Simulink.Parameter
  Fork2MaxSpd2B.Value = 3400
  Fork2MaxSpd2B.DataType = 'uint16'
  Fork2MaxSpd2B.Dimensions = [1 1]
  Fork2PosnA = Simulink.Parameter
  Fork2PosnA.Value = 798
  Fork2PosnA.DataType = 'uint16'
  Fork2PosnA.Dimensions = [1 1]
  Fork2PosnB = Simulink.Parameter
  Fork2PosnB.Value = 228
  Fork2PosnB.DataType = 'uint16'
  Fork2PosnB.Dimensions = [1 1]
  Fork2PosnMaxSpd1A = Simulink.Parameter
  Fork2PosnMaxSpd1A.Value = 540
  Fork2PosnMaxSpd1A.DataType = 'uint16'
  Fork2PosnMaxSpd1A.Dimensions = [1 1]
  Fork2PosnMaxSpd1B = Simulink.Parameter
  Fork2PosnMaxSpd1B.Value = 460
  Fork2PosnMaxSpd1B.DataType = 'uint16'
  Fork2PosnMaxSpd1B.Dimensions = [1 1]
  Fork2PosnMaxSpd2A = Simulink.Parameter
  Fork2PosnMaxSpd2A.Value = 700
  Fork2PosnMaxSpd2A.DataType = 'uint16'
  Fork2PosnMaxSpd2A.Dimensions = [1 1]
  Fork2PosnMaxSpd2B = Simulink.Parameter
  Fork2PosnMaxSpd2B.Value = 300
  Fork2PosnMaxSpd2B.DataType = 'uint16'
  Fork2PosnMaxSpd2B.Dimensions = [1 1]
  Fork2PosnNeut = Simulink.Parameter
  Fork2PosnNeut.Value = 495
  Fork2PosnNeut.DataType = 'uint16'
  Fork2PosnNeut.Dimensions = [1 1]
  Fork2PosnNeutA = Simulink.Parameter
  Fork2PosnNeutA.Value = 505
  Fork2PosnNeutA.DataType = 'uint16'
  Fork2PosnNeutA.Dimensions = [1 1]
  Fork2PosnNeutB = Simulink.Parameter
  Fork2PosnNeutB.Value = 485
  Fork2PosnNeutB.DataType = 'uint16'
  Fork2PosnNeutB.Dimensions = [1 1]
  Fork2PosnRawVal = Simulink.Signal
  Fork2PosnRawVal.Description = 'the raw value of the duty of fork 24 position pwm signal, 0-100'
  Fork2PosnRawVal.DataType = 'uint16'
  Fork2PosnRawVal.Dimensions = -1
  Fork2PosnRawVal.DimensionsMode = 'auto'
  Fork2PosnRawVal.Complexity = 'auto'
  Fork2PosnRawVal.SampleTime = -1
  Fork2PosnRawVal.SamplingMode = 'auto'
  Fork2PosnSyncA = Simulink.Parameter
  Fork2PosnSyncA.Value = 610
  Fork2PosnSyncA.DataType = 'uint16'
  Fork2PosnSyncA.Dimensions = [1 1]
  Fork2PosnSyncB = Simulink.Parameter
  Fork2PosnSyncB.Value = 390
  Fork2PosnSyncB.DataType = 'uint16'
  Fork2PosnSyncB.Dimensions = [1 1]
  Fork2PosnVal = Simulink.Signal
  Fork2PosnVal.Description = 'the value of fork 24 position, 0-100'
  Fork2PosnVal.DataType = 'uint16'
  Fork2PosnVal.Dimensions = -1
  Fork2PosnVal.DimensionsMode = 'auto'
  Fork2PosnVal.Complexity = 'auto'
  Fork2PosnVal.SampleTime = -1
  Fork2PosnVal.SamplingMode = 'auto'
  Fork2SyncTar = Simulink.Parameter
  Fork2SyncTar.Value = 20
  Fork2SyncTar.DataType = 'uint16'
  Fork2SyncTar.Dimensions = [1 1]
  Fork3A = Simulink.Parameter
  Fork3A.Value = 10
  Fork3A.DataType = 'uint8'
  Fork3A.Dimensions = [1 1]
  Fork3Act = Simulink.Signal
  Fork3Act.DataType = 'uint8'
  Fork3Act.Dimensions = -1
  Fork3Act.DimensionsMode = 'auto'
  Fork3Act.Complexity = 'auto'
  Fork3Act.SampleTime = -1
  Fork3Act.SamplingMode = 'auto'
  Fork3B = Simulink.Parameter
  Fork3B.Value = 5
  Fork3B.DataType = 'uint8'
  Fork3B.Dimensions = [1 1]
  Fork3DeltaSpdTar = Simulink.Parameter
  Fork3DeltaSpdTar.Value = 20
  Fork3DeltaSpdTar.DataType = 'uint16'
  Fork3DeltaSpdTar.Dimensions = [1 1]
  Fork3MaxSpd1A = Simulink.Parameter
  Fork3MaxSpd1A.Value = 4400
  Fork3MaxSpd1A.DataType = 'uint16'
  Fork3MaxSpd1A.Dimensions = [1 1]
  Fork3MaxSpd1B = Simulink.Parameter
  Fork3MaxSpd1B.Value = 4400
  Fork3MaxSpd1B.DataType = 'uint16'
  Fork3MaxSpd1B.Dimensions = [1 1]
  Fork3MaxSpd2A = Simulink.Parameter
  Fork3MaxSpd2A.Value = 3400
  Fork3MaxSpd2A.DataType = 'uint16'
  Fork3MaxSpd2A.Dimensions = [1 1]
  Fork3MaxSpd2B = Simulink.Parameter
  Fork3MaxSpd2B.Value = 3400
  Fork3MaxSpd2B.DataType = 'uint16'
  Fork3MaxSpd2B.Dimensions = [1 1]
  Fork3PosnA = Simulink.Parameter
  Fork3PosnA.Value = 820
  Fork3PosnA.DataType = 'uint16'
  Fork3PosnA.Dimensions = [1 1]
  Fork3PosnB = Simulink.Parameter
  Fork3PosnB.Value = 218
  Fork3PosnB.DataType = 'uint16'
  Fork3PosnB.Dimensions = [1 1]
  Fork3PosnMaxSpd1A = Simulink.Parameter
  Fork3PosnMaxSpd1A.Value = 560
  Fork3PosnMaxSpd1A.DataType = 'uint16'
  Fork3PosnMaxSpd1A.Dimensions = [1 1]
  Fork3PosnMaxSpd1B = Simulink.Parameter
  Fork3PosnMaxSpd1B.Value = 480
  Fork3PosnMaxSpd1B.DataType = 'uint16'
  Fork3PosnMaxSpd1B.Dimensions = [1 1]
  Fork3PosnMaxSpd2A = Simulink.Parameter
  Fork3PosnMaxSpd2A.Value = 720
  Fork3PosnMaxSpd2A.DataType = 'uint16'
  Fork3PosnMaxSpd2A.Dimensions = [1 1]
  Fork3PosnMaxSpd2B = Simulink.Parameter
  Fork3PosnMaxSpd2B.Value = 320
  Fork3PosnMaxSpd2B.DataType = 'uint16'
  Fork3PosnMaxSpd2B.Dimensions = [1 1]
  Fork3PosnNeut = Simulink.Parameter
  Fork3PosnNeut.Value = 515
  Fork3PosnNeut.DataType = 'uint16'
  Fork3PosnNeut.Dimensions = [1 1]
  Fork3PosnNeutA = Simulink.Parameter
  Fork3PosnNeutA.Value = 525
  Fork3PosnNeutA.DataType = 'uint16'
  Fork3PosnNeutA.Dimensions = [1 1]
  Fork3PosnNeutB = Simulink.Parameter
  Fork3PosnNeutB.Value = 505
  Fork3PosnNeutB.DataType = 'uint16'
  Fork3PosnNeutB.Dimensions = [1 1]
  Fork3PosnRawVal = Simulink.Signal
  Fork3PosnRawVal.Description = 'the raw value of the duty of fork N5 position pwm signal, 0-100'
  Fork3PosnRawVal.DataType = 'uint16'
  Fork3PosnRawVal.Dimensions = -1
  Fork3PosnRawVal.DimensionsMode = 'auto'
  Fork3PosnRawVal.Complexity = 'auto'
  Fork3PosnRawVal.SampleTime = -1
  Fork3PosnRawVal.SamplingMode = 'auto'
  Fork3PosnSyncA = Simulink.Parameter
  Fork3PosnSyncA.Value = 630
  Fork3PosnSyncA.DataType = 'uint16'
  Fork3PosnSyncA.Dimensions = [1 1]
  Fork3PosnSyncB = Simulink.Parameter
  Fork3PosnSyncB.Value = 410
  Fork3PosnSyncB.DataType = 'uint16'
  Fork3PosnSyncB.Dimensions = [1 1]
  Fork3PosnVal = Simulink.Signal
  Fork3PosnVal.Description = 'the value of fork N5 position, 0-100'
  Fork3PosnVal.DataType = 'uint16'
  Fork3PosnVal.Dimensions = -1
  Fork3PosnVal.DimensionsMode = 'auto'
  Fork3PosnVal.Complexity = 'auto'
  Fork3PosnVal.SampleTime = -1
  Fork3PosnVal.SamplingMode = 'auto'
  Fork3SyncTar = Simulink.Parameter
  Fork3SyncTar.Value = 20
  Fork3SyncTar.DataType = 'uint16'
  Fork3SyncTar.Dimensions = [1 1]
  Fork4A = Simulink.Parameter
  Fork4A.Value = 6
  Fork4A.DataType = 'uint8'
  Fork4A.Dimensions = [1 1]
  Fork4Act = Simulink.Signal
  Fork4Act.DataType = 'uint8'
  Fork4Act.Dimensions = -1
  Fork4Act.DimensionsMode = 'auto'
  Fork4Act.Complexity = 'auto'
  Fork4Act.SampleTime = -1
  Fork4Act.SamplingMode = 'auto'
  Fork4B = Simulink.Parameter
  Fork4B.Value = 7
  Fork4B.DataType = 'uint8'
  Fork4B.Dimensions = [1 1]
  Fork4DeltaSpdTar = Simulink.Parameter
  Fork4DeltaSpdTar.Value = 20
  Fork4DeltaSpdTar.DataType = 'uint16'
  Fork4DeltaSpdTar.Dimensions = [1 1]
  Fork4MaxSpd1A = Simulink.Parameter
  Fork4MaxSpd1A.Value = 4400
  Fork4MaxSpd1A.DataType = 'uint16'
  Fork4MaxSpd1A.Dimensions = [1 1]
  Fork4MaxSpd1B = Simulink.Parameter
  Fork4MaxSpd1B.Value = 4400
  Fork4MaxSpd1B.DataType = 'uint16'
  Fork4MaxSpd1B.Dimensions = [1 1]
  Fork4MaxSpd2A = Simulink.Parameter
  Fork4MaxSpd2A.Value = 3400
  Fork4MaxSpd2A.DataType = 'uint16'
  Fork4MaxSpd2A.Dimensions = [1 1]
  Fork4MaxSpd2B = Simulink.Parameter
  Fork4MaxSpd2B.Value = 3400
  Fork4MaxSpd2B.DataType = 'uint16'
  Fork4MaxSpd2B.Dimensions = [1 1]
  Fork4PosnA = Simulink.Parameter
  Fork4PosnA.Value = 810
  Fork4PosnA.DataType = 'uint16'
  Fork4PosnA.Dimensions = [1 1]
  Fork4PosnB = Simulink.Parameter
  Fork4PosnB.Value = 224
  Fork4PosnB.DataType = 'uint16'
  Fork4PosnB.Dimensions = [1 1]
  Fork4PosnMaxSpd1A = Simulink.Parameter
  Fork4PosnMaxSpd1A.Value = 560
  Fork4PosnMaxSpd1A.DataType = 'uint16'
  Fork4PosnMaxSpd1A.Dimensions = [1 1]
  Fork4PosnMaxSpd1B = Simulink.Parameter
  Fork4PosnMaxSpd1B.Value = 480
  Fork4PosnMaxSpd1B.DataType = 'uint16'
  Fork4PosnMaxSpd1B.Dimensions = [1 1]
  Fork4PosnMaxSpd2A = Simulink.Parameter
  Fork4PosnMaxSpd2A.Value = 720
  Fork4PosnMaxSpd2A.DataType = 'uint16'
  Fork4PosnMaxSpd2A.Dimensions = [1 1]
  Fork4PosnMaxSpd2B = Simulink.Parameter
  Fork4PosnMaxSpd2B.Value = 320
  Fork4PosnMaxSpd2B.DataType = 'uint16'
  Fork4PosnMaxSpd2B.Dimensions = [1 1]
  Fork4PosnNeut = Simulink.Parameter
  Fork4PosnNeut.Value = 513
  Fork4PosnNeut.DataType = 'uint16'
  Fork4PosnNeut.Dimensions = [1 1]
  Fork4PosnNeutA = Simulink.Parameter
  Fork4PosnNeutA.Value = 523
  Fork4PosnNeutA.DataType = 'uint16'
  Fork4PosnNeutA.Dimensions = [1 1]
  Fork4PosnNeutB = Simulink.Parameter
  Fork4PosnNeutB.Value = 503
  Fork4PosnNeutB.DataType = 'uint16'
  Fork4PosnNeutB.Dimensions = [1 1]
  Fork4PosnRawVal = Simulink.Signal
  Fork4PosnRawVal.Description = 'the raw value of the duty of fork 6R position pwm signal, 0-100'
  Fork4PosnRawVal.DataType = 'uint16'
  Fork4PosnRawVal.Dimensions = -1
  Fork4PosnRawVal.DimensionsMode = 'auto'
  Fork4PosnRawVal.Complexity = 'auto'
  Fork4PosnRawVal.SampleTime = -1
  Fork4PosnRawVal.SamplingMode = 'auto'
  Fork4PosnSyncA = Simulink.Parameter
  Fork4PosnSyncA.Value = 630
  Fork4PosnSyncA.DataType = 'uint16'
  Fork4PosnSyncA.Dimensions = [1 1]
  Fork4PosnSyncB = Simulink.Parameter
  Fork4PosnSyncB.Value = 410
  Fork4PosnSyncB.DataType = 'uint16'
  Fork4PosnSyncB.Dimensions = [1 1]
  Fork4PosnVal = Simulink.Signal
  Fork4PosnVal.Description = 'the value of fork 6R position, 0-100'
  Fork4PosnVal.DataType = 'uint16'
  Fork4PosnVal.Dimensions = -1
  Fork4PosnVal.DimensionsMode = 'auto'
  Fork4PosnVal.Complexity = 'auto'
  Fork4PosnVal.SampleTime = -1
  Fork4PosnVal.SamplingMode = 'auto'
  Fork4SyncTar = Simulink.Parameter
  Fork4SyncTar.Value = 20
  Fork4SyncTar.DataType = 'uint16'
  Fork4SyncTar.Dimensions = [1 1]
  FrntWhlRd = Simulink.Parameter
  FrntWhlRd.Value = 346
  FrntWhlRd.DataType = 'uint16'
  FrntWhlRd.Dimensions = [1 1]
  GearIdx = Simulink.Parameter
  GearIdx.Value = [1 2 3 4 5]
  GearIdx.DataType = 'uint8'
  GearIdx.Dimensions = [1 5]
  GearMax = Simulink.Parameter
  GearMax.Value = 6
  GearMax.DataType = 'uint8'
  GearMax.Dimensions = [1 1]
  GearRat = Simulink.Parameter
  GearRat.Value = [325 188 121 90 103 79 433]
  GearRat.DataType = 'uint16'
  GearRat.Dimensions = [1 7]
  Launch_Engage_Fuzzy : object (value not decoded)
  LnchEngmtFzzy = Simulink.LookupTable
  LnchEngmtFzzy.Table = Simulink.lookuptable.Table
  LnchEngmtFzzy.Table.Value = reshape([2 3 2 3 3 9 13 30 44 47 3 3 3 11 12 12 13 141 148 154 2 3 2 10 13 14 14 133 157 160 3 12 12 12 13 40 43 118 180 199 2 11 13 14 14 37 45 116 208 268 3 3 3 3 3 10 13 139 146 152 3 12 12 12 12 37 42 115 148 154 3 11 11 11 13 39 43 114 150 168 3 12 12 40 42 138 147 150 180 199 3 11 14 42 43 137 148 154 192 256 2 3 2 3 3 9 13 132 156 159 3 12 12 12 12 37 42 113 150 167 2 11 13 13 13 37 45 109 154 161 3 12 14 42 43 136 150 155 184 199 2 11 13 41 45 133 155 160 204 267 3 11 10 10 10 38 39 118 153 165 3 12 12 40 40 141 143 148 166 187 3 11 13 41 41 141 142 149 170 180 11 40 42 43 43 136 150 156 185 199 10 40 40 41 46 138 156 167 207 261 3 11 13 13 13 36 44 109 153 162 3 12 13 41 42 135 149 154 183 199 3 11 13 41 45 132 154 160 200 239 12 41 43 43 47 141 157 166 196 224 13 42 45 46 45 135 156 164 207 264 3 11 13 14 14 37 45 112 155 162 3 12 14 43 43 136 150 156 185 199 3 11 13 41 45 135 156 164 207 264 12 41 43 136 141 158 168 178 203 254 14 43 46 138 135 148 164 169 207 264 3 11 13 14 14 38 45 115 155 165 3 12 14 43 43 136 150 156 185 199 3 11 13 41 46 138 156 167 207 261 12 41 43 145 151 162 189 199 203 254 14 43 47 146 156 164 211 223 216 261 2 11 13 14 14 37 45 110 155 161 8 12 14 122 113 140 152 156 185 199 7 11 13 118 109 138 159 163 207 267 12 41 43 145 151 162 189 199 203 254 14 43 46 146 157 169 223 267 256 267 3 11 14 14 14 39 45 120 155 168 12 12 14 152 149 157 181 186 185 199 12 12 14 151 153 163 196 207 207 256 12 41 43 145 153 164 192 203 203 254 14 43 48 150 162 176 216 256 256 256 2 11 13 14 14 37 45 110 155 160 12 12 14 158 157 163 186 199 185 199 13 14 14 155 157 169 223 267 256 268 14 43 43 145 161 178 212 254 254 254 13 43 46 146 157 169 223 267 256 268], [10 5 10])
  LnchEngmtFzzy.Table.Dimensions = [10 5 10]
  LnchEngmtFzzy.Table.DataType = 'uint16'
  LnchEngmtFzzy.Table.FieldName = 'Table'
  LnchEngmtFzzy.Breakpoints(1) = Simulink.lookuptable.Breakpoint
  LnchEngmtFzzy.Breakpoints(1).Value = [0 11 22 33 44 56 67 78 89 100]
  LnchEngmtFzzy.Breakpoints(1).TunableSizeName = 'N1'
  LnchEngmtFzzy.Breakpoints(1).Dimensions = [1 10]
  LnchEngmtFzzy.Breakpoints(1).DataType = 'int16'
  LnchEngmtFzzy.Breakpoints(1).FieldName = 'BP1'
  LnchEngmtFzzy.Breakpoints(2) = Simulink.lookuptable.Breakpoint
  LnchEngmtFzzy.Breakpoints(2).Value = [-1000 -500 0 500 1000]
  LnchEngmtFzzy.Breakpoints(2).TunableSizeName = 'N2'
  LnchEngmtFzzy.Breakpoints(2).Dimensions = [1 5]
  LnchEngmtFzzy.Breakpoints(2).DataType = 'int16'
  LnchEngmtFzzy.Breakpoints(2).FieldName = 'BP2'
  LnchEngmtFzzy.Breakpoints(3) = Simulink.lookuptable.Breakpoint
  LnchEngmtFzzy.Breakpoints(3).Value = [0 11 22 33 44 56 67 78 89 100]
  LnchEngmtFzzy.Breakpoints(3).TunableSizeName = 'N3'
  LnchEngmtFzzy.Breakpoints(3).Dimensions = [1 10]
  LnchEngmtFzzy.Breakpoints(3).DataType = 'int16'
  LnchEngmtFzzy.Breakpoints(3).FieldName = 'BP3'
  LnchEngmtFzzy.SupportTunableSize = 0
  LnchEngmtFzzy.StructTypeInfo = Simulink.lookuptable.StructTypeInfo
  LnchEngmtFzzy.StructTypeInfo.Name = 'LnchEngmtFzzyStruct'
  LnchEngmtFzzy.StructTypeInfo.DataScope = 'Auto'
  LubeSolnIRawVal = Simulink.Signal
  LubeSolnIRawVal.DataType = 'uint16'
  LubeSolnIRawVal.Dimensions = -1
  LubeSolnIRawVal.DimensionsMode = 'auto'
  LubeSolnIRawVal.Complexity = 'auto'
  LubeSolnIRawVal.SampleTime = -1
  LubeSolnIRawVal.SamplingMode = 'auto'
  LubeSolnIReq : Simulink.Signal (value not decoded)
  LubeSolnIVal : Simulink.Signal (value not decoded)
  LubeSolnLineI : Simulink.Parameter (value not decoded)
  LubeSolnLineP : Simulink.Parameter (value not decoded)
  LubeSolnPwm : Simulink.Signal (value not decoded)
  MaiLineSolnIRawVal : Simulink.Signal (value not decoded)
  MaiLineSolnIReq : Simulink.Signal (value not decoded)
  MaiLineSolnIVal : Simulink.Signal (value not decoded)
  MaiLineSolnLineI : Simulink.Parameter (value not decoded)
  MaiLineSolnLineP : Simulink.Parameter (value not decoded)
  MaiLineSolnPwm : Simulink.Signal (value not decoded)
  OddCluPRawVal : Simulink.Signal (value not decoded)
  OddCluPVal : Simulink.Signal (value not decoded)
  OddInpSpdRawVal : Simulink.Signal (value not decoded)
  OddInpSpdVal : Simulink.Signal (value not decoded)
  OutpSpdRawVal : Simulink.Signal (value not decoded)
  OutpSpdVal : Simulink.Signal (value not decoded)
  PsnsrLineP : Simulink.Parameter (value not decoded)
  PsnsrLineV : Simulink.Parameter (value not decoded)
  SftLvrCanVal : Simulink.Signal (value not decoded)
  SftLvrCfm : Simulink.Signal (value not decoded)
  SftLvrVal : Simulink.Signal (value not decoded)
  Shaft1GearAct : Simulink.Signal (value not decoded)
  Shaft1GearReq : Simulink.Signal (value not decoded)
  Shaft2GearAct : Simulink.Signal (value not decoded)
  Shaft2GearReq : Simulink.Signal (value not decoded)
  ShiftMux1SwtReq : Simulink.Signal (value not decoded)
  ShiftMux2SwtReq : Simulink.Signal (value not decoded)
  ShiftSdlEcoDwnSeln : Simulink.Parameter (value not decoded)
  ShiftSdlEcoDwnShift : Simulink.Parameter (value not decoded)
  ShiftSdlEcoUpSeln : Simulink.Parameter (value not decoded)
  ShiftSdlEcoUpShift : Simulink.Parameter (value not decoded)
  ShiftSdlPwrDwnSeln : Simulink.Parameter (value not decoded)
  ShiftSdlPwrDwnShift : Simulink.Parameter (value not decoded)
  ShiftSdlPwrUpSeln : Simulink.Parameter (value not decoded)
  ShiftSdlPwrUpShift : Simulink.Parameter (value not decoded)
  ShiftSdlSACDwnSeln : Simulink.Parameter (value not decoded)
  ShiftSdlSACDwnShift : Simulink.Parameter (value not decoded)
  ShiftSdlSACUpSeln : Simulink.Parameter (value not decoded)
  ShiftSdlSACUpShift : Simulink.Parameter (value not decoded)
  ShiftSdlThrPedlIdx : Simulink.Parameter (value not decoded)
  ShiftSoln1IRawVal : Simulink.Signal (value not decoded)
  ShiftSoln1IReq : Simulink.Signal (value not decoded)
  ShiftSoln1IVal : Simulink.Signal (value not decoded)
  ShiftSoln1LineI : Simulink.Parameter (value not decoded)
  ShiftSoln1LineP : Simulink.Parameter (value not decoded)
  ShiftSoln1Pwm : Simulink.Signal (value not decoded)
  ShiftSoln2IRawVal : Simulink.Signal (value not decoded)
  ShiftSoln2IReq : Simulink.Signal (value not decoded)
  ShiftSoln2IVal : Simulink.Signal (value not decoded)
  ShiftSoln2LineI : Simulink.Parameter (value not decoded)
  ShiftSoln2LineP : Simulink.Parameter (value not decoded)
  ShiftSoln2Pwm : Simulink.Signal (value not decoded)
  SolnOutpTRawVal : Simulink.Signal (value not decoded)
  SolnOutpTVal : Simulink.Signal (value not decoded)
  TSnsr1LineR : Simulink.Parameter (value not decoded)
  TSnsr2LineR : Simulink.Parameter (value not decoded)
  TrsmNrGearAct : Simulink.Signal (value not decoded)
  TrsmNrGearReq : Simulink.Signal (value not decoded)
  TrsmNrPreGearAct : Simulink.Signal (value not decoded)
  TrsmNrPreGearReq : Simulink.Signal (value not decoded)
  Tsnsr1LineT : Simulink.Parameter (value not decoded)
  Tsnsr2LineT : Simulink.Parameter (value not decoded)
  VehSpdCanVal : Simulink.Signal (value not decoded)
  VehSpdTrsmEstimd : Simulink.Signal (value not decoded)
  VehSpdVal : Simulink.Signal (value not decoded)
  VlvBodyTRawVal : Simulink.Signal (value not decoded)
  VlvBodyTVal : Simulink.Signal (value not decoded)
undefined symbols (not defined in the file or in its folder): in1, out1
libraries: simulink x44, fuzblock x3
(part 1 of 10)
settings Model: Creator=SHAW  LastModifiedBy=DELL
settings DataIOCC: LimitDataPoints=on  SaveFormat=Array  ReturnWorkspaceOutputs=off
settings OptimizationCC: LifeSpan=inf
settings DebuggingCC: SolverPrmCheckMsg=warning  SFUnexpectedBacktrackingDiag=warning  SFNoUnconditionalDefaultTransitionDiag=warning  SFExecutionAtInitializationDiag=none  ArithmeticOperatorsInVariantConditions=warning
settings HardwareCC: ProdBitPerInt=16  ProdBitPerPointer=16  ProdBitPerSizeT=16  ProdBitPerPtrDiffT=16  ProdLargestAtomicFloat=None  ProdIntDivRoundTo=Undefined  ProdEndianess=BigEndian  ProdWordSize=16  ProdHWDeviceType=Freescale->S12x
settings ModelReferenceCC: PropagateSignalLabelsOutOfModel=off
settings SFSimCC: SimUseLocalCustomCode=off  CustomCodeUndefinedFunction=UseInterfaceOnly
settings RTWCC: RTWUseLocalCustomCode=off
settings CodeAppCC: StateflowObjectComments=on
settings GRTTargetCC: TargetLangStandard=C89/C90 (ANSI)
settings ConfigComp: CovMetricSettings=dw  CovHtmlReporting=on  CovSaveCumulativeToWorkspaceVar=on  CovSaveSingleToWorkspaceVar=on  CovExternalEMLEnable=off  CovSFcnEnable=off

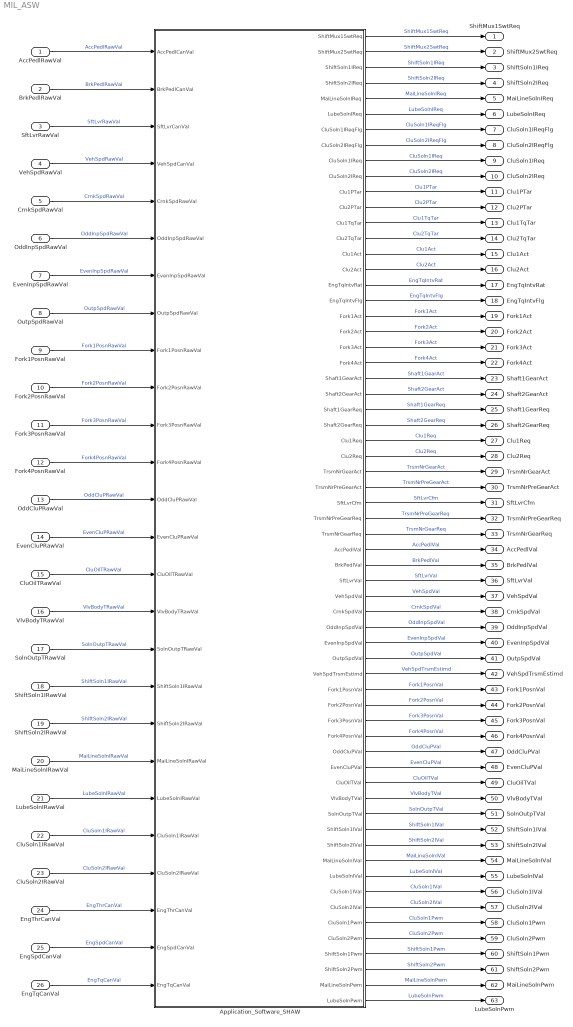
== system MIL_ASW ==
  AccPedlRawVal : Inport  OutDataTypeStr=uint8
  BrkPedlRawVal : Inport  Port=2  OutDataTypeStr=uint8
  SftLvrRawVal : Inport  Port=3  OutDataTypeStr=uint8
  VehSpdRawVal : Inport  Port=4  OutDataTypeStr=uint16
  CrnkSpdRawVal : Inport  Port=5  OutDataTypeStr=uint16
  OddInpSpdRawVal : Inport  Port=6  OutDataTypeStr=uint16
  EvenInpSpdRawVal : Inport  Port=7  OutDataTypeStr=uint16
  OutpSpdRawVal : Inport  Port=8  OutDataTypeStr=uint16
  Fork1PosnRawVal : Inport  Port=9  OutDataTypeStr=uint16
  Fork2PosnRawVal : Inport  Port=10  OutDataTypeStr=uint16
  Fork3PosnRawVal : Inport  Port=11  OutDataTypeStr=uint16
  Fork4PosnRawVal : Inport  Port=12  OutDataTypeStr=uint16
  OddCluPRawVal : Inport  Port=13  OutDataTypeStr=uint16
  EvenCluPRawVal : Inport  Port=14  OutDataTypeStr=uint16
  CluOilTRawVal : Inport  Port=15  OutDataTypeStr=uint16
  VlvBodyTRawVal : Inport  Port=16  OutDataTypeStr=uint16
  SolnOutpTRawVal : Inport  Port=17  OutDataTypeStr=uint16
  ShiftSoln1IRawVal : Inport  Port=18  OutDataTypeStr=uint16
  ShiftSoln2IRawVal : Inport  Port=19  OutDataTypeStr=uint16
  MaiLineSolnIRawVal : Inport  Port=20  OutDataTypeStr=uint16
  LubeSolnIRawVal : Inport  Port=21  OutDataTypeStr=uint16
  CluSoln1IRawVal : Inport  Port=22  OutDataTypeStr=uint16
  CluSoln2IRawVal : Inport  Port=23  OutDataTypeStr=uint16
  EngThrCanVal : Inport  Port=24
  EngSpdCanVal : Inport  Port=25
  EngTqCanVal : Inport  Port=26
  Application_Software_SHAW : Subsystem
  ShiftMux1SwtReq : Outport  VectorParamsAs1DForOutWhenUnconnected=off
  ShiftMux2SwtReq : Outport  Port=2  VectorParamsAs1DForOutWhenUnconnected=off
  ShiftSoln1IReq : Outport  Port=3  VectorParamsAs1DForOutWhenUnconnected=off
  ShiftSoln2IReq : Outport  Port=4  VectorParamsAs1DForOutWhenUnconnected=off
  MaiLineSolnIReq : Outport  Port=5  VectorParamsAs1DForOutWhenUnconnected=off
  LubeSolnIReq : Outport  Port=6  VectorParamsAs1DForOutWhenUnconnected=off
  CluSoln1IReqFlg : Outport  Port=7  VectorParamsAs1DForOutWhenUnconnected=off
  CluSoln2IReqFlg : Outport  Port=8  VectorParamsAs1DForOutWhenUnconnected=off
  CluSoln1IReq : Outport  Port=9  VectorParamsAs1DForOutWhenUnconnected=off
  CluSoln2IReq : Outport  Port=10  VectorParamsAs1DForOutWhenUnconnected=off
  Clu1PTar : Outport  Port=11  OutDataTypeStr=uint16  VectorParamsAs1DForOutWhenUnconnected=off
  Clu2PTar : Outport  Port=12  OutDataTypeStr=uint16  VectorParamsAs1DForOutWhenUnconnected=off
  Clu1TqTar : Outport  Port=13  VectorParamsAs1DForOutWhenUnconnected=off
  Clu2TqTar : Outport  Port=14  VectorParamsAs1DForOutWhenUnconnected=off
  Clu1Act : Outport  Port=15  VectorParamsAs1DForOutWhenUnconnected=off
  Clu2Act : Outport  Port=16  VectorParamsAs1DForOutWhenUnconnected=off
  EngTqIntvRat : Outport  Port=17  VectorParamsAs1DForOutWhenUnconnected=off
  EngTqIntvFlg : Outport  Port=18  VectorParamsAs1DForOutWhenUnconnected=off
  Fork1Act : Outport  Port=19  VectorParamsAs1DForOutWhenUnconnected=off
  Fork2Act : Outport  Port=20  VectorParamsAs1DForOutWhenUnconnected=off
  Fork3Act : Outport  Port=21  VectorParamsAs1DForOutWhenUnconnected=off
  Fork4Act : Outport  Port=22  VectorParamsAs1DForOutWhenUnconnected=off
  Shaft1GearAct : Outport  Port=23  VectorParamsAs1DForOutWhenUnconnected=off
  Shaft2GearAct : Outport  Port=24  VectorParamsAs1DForOutWhenUnconnected=off
  Shaft1GearReq : Outport  Port=25  VectorParamsAs1DForOutWhenUnconnected=off
  Shaft2GearReq : Outport  Port=26  VectorParamsAs1DForOutWhenUnconnected=off
  Clu1Req : Outport  Port=27  VectorParamsAs1DForOutWhenUnconnected=off
  Clu2Req : Outport  Port=28  VectorParamsAs1DForOutWhenUnconnected=off
  TrsmNrGearAct : Outport  Port=29  VectorParamsAs1DForOutWhenUnconnected=off
  TrsmNrPreGearAct : Outport  Port=30  VectorParamsAs1DForOutWhenUnconnected=off
  SftLvrCfm : Outport  Port=31  VectorParamsAs1DForOutWhenUnconnected=off
  TrsmNrPreGearReq : Outport  Port=32  OutDataTypeStr=uint8  VectorParamsAs1DForOutWhenUnconnected=off
  TrsmNrGearReq : Outport  Port=33  OutDataTypeStr=uint8  VectorParamsAs1DForOutWhenUnconnected=off
  AccPedlVal : Outport  Port=34  VectorParamsAs1DForOutWhenUnconnected=off
  BrkPedlVal : Outport  Port=35  OutDataTypeStr=uint8  VectorParamsAs1DForOutWhenUnconnected=off
  SftLvrVal : Outport  Port=36  OutDataTypeStr=uint8  VectorParamsAs1DForOutWhenUnconnected=off
  VehSpdVal : Outport  Port=37  VectorParamsAs1DForOutWhenUnconnected=off
  CrnkSpdVal : Outport  Port=38  VectorParamsAs1DForOutWhenUnconnected=off
  OddInpSpdVal : Outport  Port=39  VectorParamsAs1DForOutWhenUnconnected=off
  EvenInpSpdVal : Outport  Port=40  VectorParamsAs1DForOutWhenUnconnected=off
  OutpSpdVal : Outport  Port=41  VectorParamsAs1DForOutWhenUnconnected=off
  VehSpdTrsmEstimd : Outport  Port=42  VectorParamsAs1DForOutWhenUnconnected=off
  Fork1PosnVal : Outport  Port=43  VectorParamsAs1DForOutWhenUnconnected=off
  Fork2PosnVal : Outport  Port=44  VectorParamsAs1DForOutWhenUnconnected=off
  Fork3PosnVal : Outport  Port=45  VectorParamsAs1DForOutWhenUnconnected=off
  Fork4PosnVal : Outport  Port=46  VectorParamsAs1DForOutWhenUnconnected=off
  OddCluPVal : Outport  Port=47  VectorParamsAs1DForOutWhenUnconnected=off
  EvenCluPVal : Outport  Port=48  VectorParamsAs1DForOutWhenUnconnected=off
  CluOilTVal : Outport  Port=49  VectorParamsAs1DForOutWhenUnconnected=off
  VlvBodyTVal : Outport  Port=50  VectorParamsAs1DForOutWhenUnconnected=off
  SolnOutpTVal : Outport  Port=51  VectorParamsAs1DForOutWhenUnconnected=off
  ShiftSoln1IVal : Outport  Port=52  VectorParamsAs1DForOutWhenUnconnected=off
  ShiftSoln2IVal : Outport  Port=53  VectorParamsAs1DForOutWhenUnconnected=off
  MaiLineSolnIVal : Outport  Port=54  VectorParamsAs1DForOutWhenUnconnected=off
  LubeSolnIVal : Outport  Port=55  VectorParamsAs1DForOutWhenUnconnected=off
  CluSoln1IVal : Outport  Port=56  VectorParamsAs1DForOutWhenUnconnected=off
  CluSoln2IVal : Outport  Port=57  VectorParamsAs1DForOutWhenUnconnected=off
  CluSoln1Pwm : Outport  Port=58  VectorParamsAs1DForOutWhenUnconnected=off
  CluSoln2Pwm : Outport  Port=59  VectorParamsAs1DForOutWhenUnconnected=off
  ShiftSoln1Pwm : Outport  Port=60  VectorParamsAs1DForOutWhenUnconnected=off
  ShiftSoln2Pwm : Outport  Port=61  VectorParamsAs1DForOutWhenUnconnected=off
  MaiLineSolnPwm : Outport  Port=62  VectorParamsAs1DForOutWhenUnconnected=off
  LubeSolnPwm : Outport  Port=63  VectorParamsAs1DForOutWhenUnconnected=off
  wires:
  Application_Software_SHAW/26(Shaft2GearReq) -> Shaft2GearReq/1  "Shaft2GearReq"
  Application_Software_SHAW/14(Clu2TqTar) -> Clu2TqTar/1  "Clu2TqTar"
  Application_Software_SHAW/28(Clu2Req) -> Clu2Req/1  "Clu2Req"
  Application_Software_SHAW/22(Fork4Act) -> Fork4Act/1  "Fork4Act"
  Application_Software_SHAW/33(TrsmNrGearReq) -> TrsmNrGearReq/1  "TrsmNrGearReq"
  Application_Software_SHAW/34(AccPedlVal) -> AccPedlVal/1  "AccPedlVal"
  Application_Software_SHAW/36(SftLvrVal) -> SftLvrVal/1  "SftLvrVal"
  Application_Software_SHAW/32(TrsmNrPreGearReq) -> TrsmNrPreGearReq/1  "TrsmNrPreGearReq"
  Application_Software_SHAW/2(ShiftMux2SwtReq) -> ShiftMux2SwtReq/1  "ShiftMux2SwtReq"
  Application_Software_SHAW/20(Fork2Act) -> Fork2Act/1  "Fork2Act"
  Application_Software_SHAW/10(CluSoln2IReq) -> CluSoln2IReq/1  "CluSoln2IReq"
  Application_Software_SHAW/24(Shaft2GearAct) -> Shaft2GearAct/1  "Shaft2GearAct"
  Application_Software_SHAW/41(OutpSpdVal) -> OutpSpdVal/1  "OutpSpdVal"
  Application_Software_SHAW/15(Clu1Act) -> Clu1Act/1  "Clu1Act"
  Application_Software_SHAW/1(ShiftMux1SwtReq) -> ShiftMux1SwtReq/1  "ShiftMux1SwtReq"
  Application_Software_SHAW/19(Fork1Act) -> Fork1Act/1  "Fork1Act"
  Application_Software_SHAW/27(Clu1Req) -> Clu1Req/1  "Clu1Req"
  Application_Software_SHAW/46(Fork4PosnVal) -> Fork4PosnVal/1  "Fork4PosnVal"
  Application_Software_SHAW/13(Clu1TqTar) -> Clu1TqTar/1  "Clu1TqTar"
  Application_Software_SHAW/38(CrnkSpdVal) -> CrnkSpdVal/1  "CrnkSpdVal"
  Application_Software_SHAW/49(CluOilTVal) -> CluOilTVal/1  "CluOilTVal"
  Application_Software_SHAW/6(LubeSolnIReq) -> LubeSolnIReq/1  "LubeSolnIReq"
  Application_Software_SHAW/11(Clu1PTar) -> Clu1PTar/1  "Clu1PTar"
  Application_Software_SHAW/4(ShiftSoln2IReq) -> ShiftSoln2IReq/1  "ShiftSoln2IReq"
  Application_Software_SHAW/35(BrkPedlVal) -> BrkPedlVal/1  "BrkPedlVal"
  Application_Software_SHAW/25(Shaft1GearReq) -> Shaft1GearReq/1  "Shaft1GearReq"
  Application_Software_SHAW/16(Clu2Act) -> Clu2Act/1  "Clu2Act"
  Application_Software_SHAW/3(ShiftSoln1IReq) -> ShiftSoln1IReq/1  "ShiftSoln1IReq"
  Application_Software_SHAW/8(CluSoln2IReqFlg) -> CluSoln2IReqFlg/1  "CluSoln2IReqFlg"
  Application_Software_SHAW/29(TrsmNrGearAct) -> TrsmNrGearAct/1  "TrsmNrGearAct"
  Application_Software_SHAW/42(VehSpdTrsmEstimd) -> VehSpdTrsmEstimd/1  "VehSpdTrsmEstimd"
  Application_Software_SHAW/44(Fork2PosnVal) -> Fork2PosnVal/1  "Fork2PosnVal"
  Application_Software_SHAW/39(OddInpSpdVal) -> OddInpSpdVal/1  "OddInpSpdVal"
  Application_Software_SHAW/50(VlvBodyTVal) -> VlvBodyTVal/1  "VlvBodyTVal"
  Application_Software_SHAW/51(SolnOutpTVal) -> SolnOutpTVal/1  "SolnOutpTVal"
  Application_Software_SHAW/48(EvenCluPVal) -> EvenCluPVal/1  "EvenCluPVal"
  Application_Software_SHAW/7(CluSoln1IReqFlg) -> CluSoln1IReqFlg/1  "CluSoln1IReqFlg"
  Application_Software_SHAW/23(Shaft1GearAct) -> Shaft1GearAct/1  "Shaft1GearAct"
  Application_Software_SHAW/45(Fork3PosnVal) -> Fork3PosnVal/1  "Fork3PosnVal"
  Application_Software_SHAW/53(ShiftSoln2IVal) -> ShiftSoln2IVal/1  "ShiftSoln2IVal"
  Application_Software_SHAW/43(Fork1PosnVal) -> Fork1PosnVal/1  "Fork1PosnVal"
  Application_Software_SHAW/47(OddCluPVal) -> OddCluPVal/1  "OddCluPVal"
  Application_Software_SHAW/52(ShiftSoln1IVal) -> ShiftSoln1IVal/1  "ShiftSoln1IVal"
  Application_Software_SHAW/54(MaiLineSolnIVal) -> MaiLineSolnIVal/1  "MaiLineSolnIVal"
  Application_Software_SHAW/55(LubeSolnIVal) -> LubeSolnIVal/1  "LubeSolnIVal"
  Application_Software_SHAW/56(CluSoln1IVal) -> CluSoln1IVal/1  "CluSoln1IVal"
  Application_Software_SHAW/57(CluSoln2IVal) -> CluSoln2IVal/1  "CluSoln2IVal"
  Application_Software_SHAW/9(CluSoln1IReq) -> CluSoln1IReq/1  "CluSoln1IReq"
  Application_Software_SHAW/17(EngTqIntvRat) -> EngTqIntvRat/1  "EngTqIntvRat"
  Application_Software_SHAW/31(SftLvrCfm) -> SftLvrCfm/1  "SftLvrCfm"
  Application_Software_SHAW/37(VehSpdVal) -> VehSpdVal/1  "VehSpdVal"
  Application_Software_SHAW/40(EvenInpSpdVal) -> EvenInpSpdVal/1  "EvenInpSpdVal"
  Application_Software_SHAW/30(TrsmNrPreGearAct) -> TrsmNrPreGearAct/1  "TrsmNrPreGearAct"
  Application_Software_SHAW/5(MaiLineSolnIReq) -> MaiLineSolnIReq/1  "MaiLineSolnIReq"
  Application_Software_SHAW/12(Clu2PTar) -> Clu2PTar/1  "Clu2PTar"
  Application_Software_SHAW/18(EngTqIntvFlg) -> EngTqIntvFlg/1  "EngTqIntvFlg"
  Application_Software_SHAW/21(Fork3Act) -> Fork3Act/1  "Fork3Act"
  VehSpdRawVal/1 -> Application_Software_SHAW/4(VehSpdCanVal)  "VehSpdRawVal"
  OutpSpdRawVal/1 -> Application_Software_SHAW/8(OutpSpdRawVal)  "OutpSpdRawVal"
  Fork1PosnRawVal/1 -> Application_Software_SHAW/9(Fork1PosnRawVal)  "Fork1PosnRawVal"
  OddInpSpdRawVal/1 -> Application_Software_SHAW/6(OddInpSpdRawVal)  "OddInpSpdRawVal"
  EvenInpSpdRawVal/1 -> Application_Software_SHAW/7(EvenInpSpdRawVal)  "EvenInpSpdRawVal"
  CluSoln1IRawVal/1 -> Application_Software_SHAW/22(CluSoln1IRawVal)  "CluSoln1IRawVal"
  Fork3PosnRawVal/1 -> Application_Software_SHAW/11(Fork3PosnRawVal)  "Fork3PosnRawVal"
  SolnOutpTRawVal/1 -> Application_Software_SHAW/17(SolnOutpTRawVal)  "SolnOutpTRawVal"
  SftLvrRawVal/1 -> Application_Software_SHAW/3(SftLvrCanVal)  "SftLvrRawVal"
  CrnkSpdRawVal/1 -> Application_Software_SHAW/5(CrnkSpdRawVal)  "CrnkSpdRawVal"
  Fork2PosnRawVal/1 -> Application_Software_SHAW/10(Fork2PosnRawVal)  "Fork2PosnRawVal"
  Fork4PosnRawVal/1 -> Application_Software_SHAW/12(Fork4PosnRawVal)  "Fork4PosnRawVal"
  MaiLineSolnIRawVal/1 -> Application_Software_SHAW/20(MaiLineSolnIRawVal)  "MaiLineSolnIRawVal"
  LubeSolnIRawVal/1 -> Application_Software_SHAW/21(LubeSolnIRawVal)  "LubeSolnIRawVal"
  CluOilTRawVal/1 -> Application_Software_SHAW/15(CluOilTRawVal)  "CluOilTRawVal"
  CluSoln2IRawVal/1 -> Application_Software_SHAW/23(CluSoln2IRawVal)  "CluSoln2IRawVal"
  OddCluPRawVal/1 -> Application_Software_SHAW/13(OddCluPRawVal)  "OddCluPRawVal"
  EvenCluPRawVal/1 -> Application_Software_SHAW/14(EvenCluPRawVal)  "EvenCluPRawVal"
  BrkPedlRawVal/1 -> Application_Software_SHAW/2(BrkPedlCanVal)  "BrkPedlRawVal"
  AccPedlRawVal/1 -> Application_Software_SHAW/1(AccPedlCanVal)  "AccPedlRawVal"
  ShiftSoln1IRawVal/1 -> Application_Software_SHAW/18(ShiftSoln1IRawVal)  "ShiftSoln1IRawVal"
  VlvBodyTRawVal/1 -> Application_Software_SHAW/16(VlvBodyTRawVal)  "VlvBodyTRawVal"
  ShiftSoln2IRawVal/1 -> Application_Software_SHAW/19(ShiftSoln2IRawVal)  "ShiftSoln2IRawVal"
  Application_Software_SHAW/58(CluSoln1Pwm) -> CluSoln1Pwm/1  "CluSoln1Pwm"
  Application_Software_SHAW/59(CluSoln2Pwm) -> CluSoln2Pwm/1  "CluSoln2Pwm"
  Application_Software_SHAW/60(ShiftSoln1Pwm) -> ShiftSoln1Pwm/1  "ShiftSoln1Pwm"
  Application_Software_SHAW/61(ShiftSoln2Pwm) -> ShiftSoln2Pwm/1  "ShiftSoln2Pwm"
  Application_Software_SHAW/62(MaiLineSolnPwm) -> MaiLineSolnPwm/1  "MaiLineSolnPwm"
  Application_Software_SHAW/63(LubeSolnPwm) -> LubeSolnPwm/1  "LubeSolnPwm"
  EngThrCanVal/1 -> Application_Software_SHAW/24(EngThrCanVal)  "EngThrCanVal"
  EngSpdCanVal/1 -> Application_Software_SHAW/25(EngSpdCanVal)  "EngSpdCanVal"
  EngTqCanVal/1 -> Application_Software_SHAW/26(EngTqCanVal)  "EngTqCanVal"
